simulink model "adaptive_cc"  (R2026a)
settings: Solver=FixedStepDiscrete  StopTime=30  FixedStep=0.1
undefined symbols (not defined in the file): DiscIntNeverNeededParam
settings Model: Creator=parth  LastModifiedBy=parth

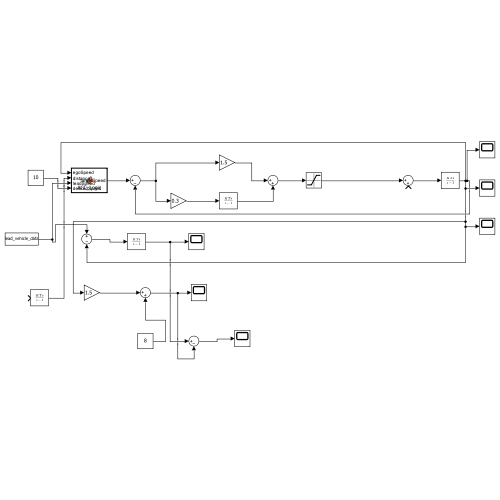
[thumbnail: Simulink's stored preview of the top-level diagram]
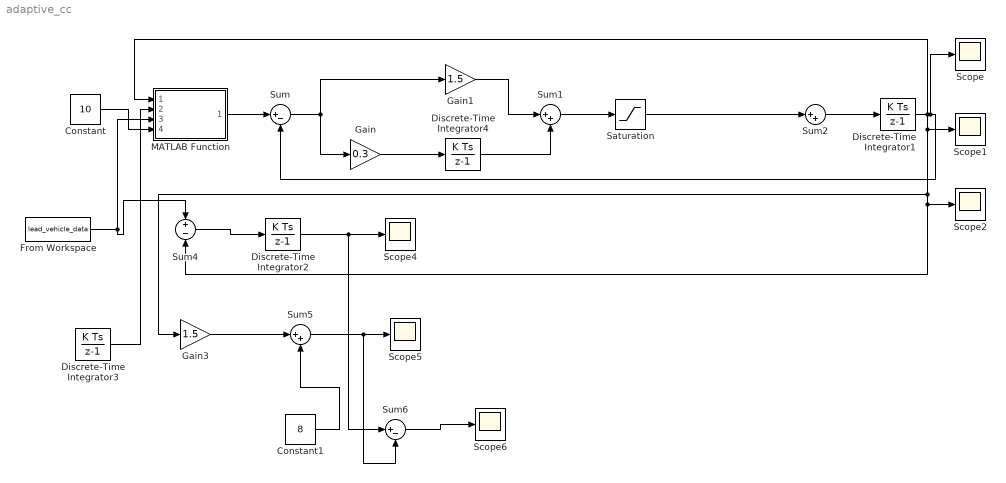
== system adaptive_cc ==
  Constant : Constant  Value=10
  Constant1 : Constant  Value=8
  Discrete-Time Integrator1 : DiscreteIntegrator  SampleTime=0.1  ICPrevOutput=DiscIntNeverNeededParam  ICPrevScaledInput=DiscIntNeverNeededParam
  Discrete-Time Integrator2 : DiscreteIntegrator  InitialCondition=30  SampleTime=0.1  ICPrevOutput=DiscIntNeverNeededParam  ICPrevScaledInput=DiscIntNeverNeededParam
  Discrete-Time Integrator3 : DiscreteIntegrator  SampleTime=-1  ICPrevOutput=DiscIntNeverNeededParam  ICPrevScaledInput=DiscIntNeverNeededParam
  Discrete-Time Integrator4 : DiscreteIntegrator  gainval=1  SampleTime=0.1  ICPrevOutput=DiscIntNeverNeededParam  ICPrevScaledInput=DiscIntNeverNeededParam
  From Workspace : FromWorkspace  VariableName=lead_vehicle_data
  Gain : Gain  Gain=0.3
  Gain1 : Gain  Gain=1.5
  Gain3 : Gain  Gain=1.5
  MATLAB Function : MATLAB Function  TreatAsAtomicUnit=on
  Saturation : Saturate  UpperLimit=3  LowerLimit=-4
  Scope{,1..2,4..6} (6 alike) : Scope
      Scope settings: ActiveDisplayYMinimum=-1  ActiveDisplayYMaximum=1
      Scope1 settings: ActiveDisplayYMinimum=-1  ActiveDisplayYMaximum=1
      Scope2 settings: ActiveDisplayYMinimum=-1  ActiveDisplayYMaximum=1  DataLoggingVariableName=ScopeData2
      Scope4 settings: ActiveDisplayYMinimum=-1  ActiveDisplayYMaximum=1  DataLoggingVariableName=ScopeData4
      Scope5 settings: ActiveDisplayYMinimum=-1  ActiveDisplayYMaximum=1  DataLoggingVariableName=ScopeData5
      Scope6 settings: ActiveDisplayYMinimum=11.012380527256404  ActiveDisplayYMaximum=98.40851201522328  DataLoggingVariableName=ScopeData6
  Sum : Sum  Inputs=|+-
  Sum1 : Sum  Inputs=|++
  Sum2 : Sum  Inputs=|++
  Sum4 : Sum  Inputs=+-
  Sum5 : Sum  Inputs=|++
  Sum6 : Sum  Inputs=|+-
  wires:
  Constant/1 -> MATLAB Function/4(desiredSpeed)
  From Workspace/1 -> Sum4/1, MATLAB Function/3(leadSpeed)
  Discrete-Time Integrator3/1 -> MATLAB Function/2(distance)
  Sum4/1 -> Discrete-Time Integrator2/1
  Discrete-Time Integrator2/1 -> Sum6/1, Scope4/1
  MATLAB Function/1(targetSpeed) -> Sum/1
  Sum/1 -> Gain1/1, Gain/1
  Gain1/1 -> Sum1/1
  Sum1/1 -> Saturation/1
  Discrete-Time Integrator1/1 -> MATLAB Function/1(egoSpeed), Sum/2, Scope/1, Sum4/2, Scope2/1, Gain3/1, Scope1/1
  Saturation/1 -> Sum2/1
  Sum2/1 -> Discrete-Time Integrator1/1
  Constant1/1 -> Sum5/2
  Sum5/1 -> Sum6/2, Scope5/1
  Sum6/1 -> Scope6/1
  Gain/1 -> Discrete-Time Integrator4/1
  Discrete-Time Integrator4/1 -> Sum1/2
  Gain3/1 -> Sum5/1

== matlab function adaptive_cc/MATLAB Function ==
  data: egoSpeed input; targetSpeed output; distance input; leadSpeed input; desiredSpeed input
function targetSpeed = ACC_Logic(egoSpeed, distance, leadSpeed, desiredSpeed)

minimumDistance = 8;
timeGap = 1.5;

safeDistance = minimumDistance + timeGap * egoSpeed;

distanceError = distance - safeDistance;

if distanceError > 10

    targetSpeed = desiredSpeed;

elseif distanceError > 0

    targetSpeed = min(desiredSpeed, leadSpeed);

elseif distanceError > -3

    targetSpeed = max(0, leadSpeed - 1);

else

    targetSpeed = max(0, leadSpeed - 2);

end
